simulink model "proc_control_node"  (R2020a)
settings: Solver=FixedStepAuto  StartTime=0.0  StopTime=inf  FixedStep=.005  RelTol=1e-3
model workspace (MAT data in the model file):
  SL_ROS_VariableLengthArrays_MaxSizes.CommonInfo.ArrayTruncateAction = 'EmitWarning'
  SL_ROS_VariableLengthArrays_MaxSizes.MsgTypeMap = containers.Map
  SL_ROS_VariableLengthArrays_MaxSizes.MsgTypeMap.serialization.keys = {}
  SL_ROS_VariableLengthArrays_MaxSizes.MsgTypeMap.serialization.values = {}
  SL_ROS_VariableLengthArrays_MaxSizes.MsgTypeMap.serialization.uniformity = 0
  SL_ROS_VariableLengthArrays_MaxSizes.MsgTypeMap.serialization.keyType = 'char'
  SL_ROS_VariableLengthArrays_MaxSizes.MsgTypeMap.serialization.valueType = 'any'
undefined symbols (not defined in the file): InitController
libraries: robotlib x6, simulink x1
settings Model: SimulationMode=accelerator  PauseTimes=1000  Creator=Lamarre  LastModifiedBy=lamarre
settings OptimizationCC: EnhancedBackFolding=on  PassReuseOutputArgsAs=Individual arguments  ZeroExternalMemoryAtStartup=off  ZeroInternalMemoryAtStartup=off  MaxStackSize=64  OptimizeBlockOrder=speed  DifferentSizesBufferReuse=on  OptimizationCustomize=off  EfficientTunableParamExpr=on
settings DebuggingCC: ParameterTunabilityLossMsg=error  FcnCallInpInsideContextMsg=warning  UnderSpecifiedDimensionMsg=warning
settings HardwareCC: ProdBitPerPointer=32  ProdBitPerSizeT=32  ProdBitPerPtrDiffT=32  ProdLargestAtomicInteger=Long  ProdWordSize=32  ProdHWDeviceType=ARM Compatible->ARM 8
settings ModelReferenceCC: ModelReferenceNumInstancesAllowed=Single
settings SFSimCC: MATLABDynamicMemAlloc=off
settings RTWCC: SystemTargetFile=ert.tlc  HardwareBoard=Robot Operating System (ROS)  TemplateMakefile=ert_default_tmf  Toolchain=Catkin  BuildConfiguration=Faster Runs  TargetLang=C++
settings CodeAppCC: ForceParamTrailComments=on  IgnoreCustomStorageClasses=off  OperatorAnnotations=on  SimulinkDataObjDesc=on  SFDataObjDesc=on  InsertBlockDesc=on
settings ERTTargetCC: SupportContinuousTime=on  SupportVariableSizeSignals=on  TargetOS=NativeThreadsExample  MultiInstanceErrorCode=Warning  RootIOFormat=Structure reference

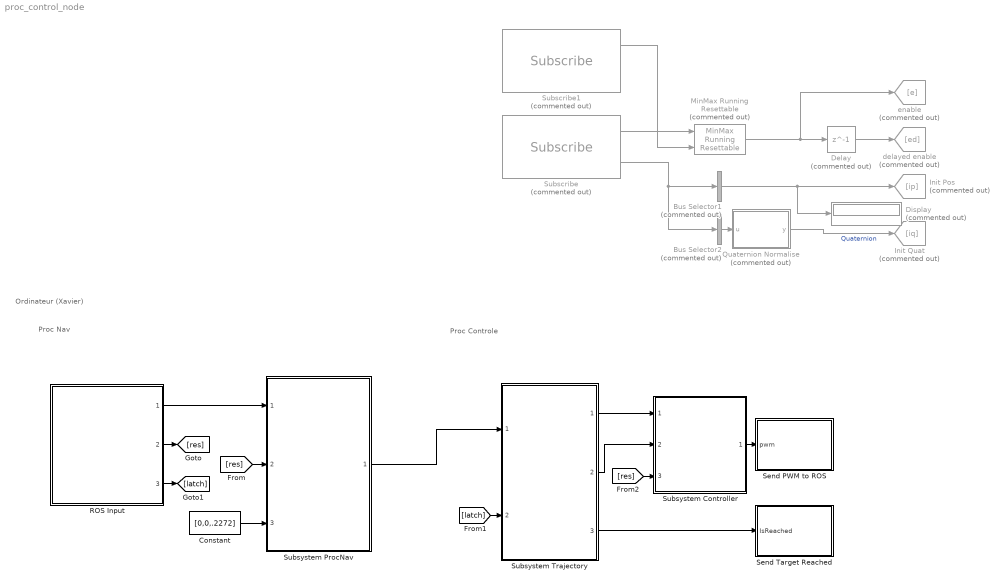
== system proc_control_node ==
  note: Proc Nav
  note: Proc Controle
  note: Ordinateur (Xavier)
  " Init Pos" : Goto  Commented=on  GotoTag=ip
  " Init Quat" : Goto  Commented=on  GotoTag=iq
  " enable" : Goto  Commented=on  GotoTag=e
  Bus Selector1 : BusSelector  Commented=on  OutputSignals=Position.X,Position.Y,Position.Z  OutputAsBus=on
  Bus Selector2 : BusSelector  Commented=on  OutputSignals=Orientation.W,Orientation.Z,Orientation.Y,Orientation.X  OutputAsBus=on
  Constant : Constant  Value=[0,0,.2272]
  Delay : Delay  Commented=on  DelayLength=1
  Display : Display  Commented=on
  MinMax Running Resettable : simulink/Math Operations/MinMax Running Resettable  Commented=on  Function=max  vinit=0.0
  Quaternion Normalise : MATLAB Function  Commented=on  TreatAsAtomicUnit=on
  ROS Input : Subsystem  ReferencedSubsystem=proc_nav_ros_input
  Send PWM to ROS : Subsystem
  "Send Target Reached " : Subsystem
  Subscribe : robotlib/Subscribe  Commented=on  topicSource=Specify your own  topic=/proc_control/start  messageType=geometry_msgs/Pose  sampleTime=-1  messageQueueLength=1
  Subscribe1 : robotlib/Subscribe  Commented=on  topicSource=Specify your own  topic=/proc_control/kill  messageType=std_msgs/Bool  sampleTime=-1  messageQueueLength=1
  Subsystem Controller : Subsystem  InitFcn=InitController;  ReferencedSubsystem=Controller
  Subsystem ProcNav : Subsystem  ReferencedSubsystem=ProcNav
  Subsystem Trajectory : Subsystem  InitFcn=|  ReferencedSubsystem=Trajectory
      | InitTrajectory
      | %trajec;
  delayed enable : Goto  Commented=on  GotoTag=ed
  wires:
  Subsystem ProcNav/1 -> Subsystem Trajectory/1
  Subsystem Trajectory/1 -> Subsystem Controller/1
  Constant/1 -> Subsystem ProcNav/3
  Subsystem Trajectory/2 -> Subsystem Controller/2
  Subsystem Trajectory/3 -> "Send Target Reached "/1(IsReached)
  MinMax Running Resettable/1 -> " enable"/1, Delay/1
  Subscribe/1 -> MinMax Running Resettable/1
  Subscribe/2 -> Bus Selector2/1, Bus Selector1/1
  Delay/1 -> delayed enable/1
  Bus Selector1/1 -> Display/1, " Init Pos"/1
  Subscribe1/1 -> MinMax Running Resettable/2
  Bus Selector2/1 -> Quaternion Normalise/1(u)
  Quaternion Normalise/1(y) -> " Init Quat"/1  "Quaternion"
  Subsystem Controller/1 -> Send PWM to ROS/1(pwm)
  ROS Input/1 -> Subsystem ProcNav/1
  ROS Input/2 -> [res]
  [res] -> Subsystem ProcNav/2
  [latch] -> Subsystem Trajectory/2
  [res] -> Subsystem Controller/3
  ROS Input/3 -> [latch]

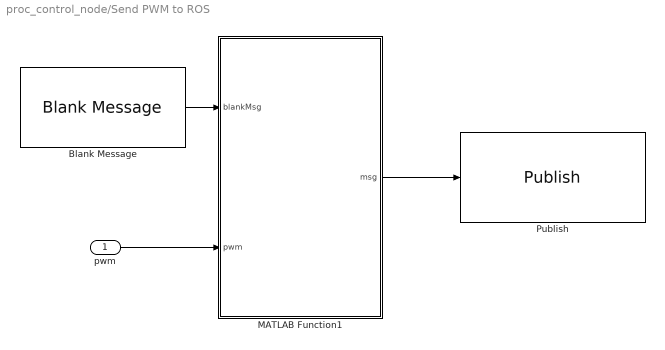
== system proc_control_node/Send PWM to ROS ==
  pwm : Inport
  Blank Message : robotlib/Blank Message  messageClass=Message  entityType=std_msgs/UInt16MultiArray  messageType=std_msgs/UInt16MultiArray  SampleTime=inf
  MATLAB Function1 : MATLAB Function  TreatAsAtomicUnit=on
  Publish : robotlib/Publish  topicSource=Specify your own  topic=/provider_thruster/thruster_pwm  messageType=std_msgs/UInt16MultiArray  messageQueueLength=1
  wires:
  MATLAB Function1/1(msg) -> Publish/1
  Blank Message/1 -> MATLAB Function1/1(blankMsg)
  pwm/1 -> MATLAB Function1/2(pwm)

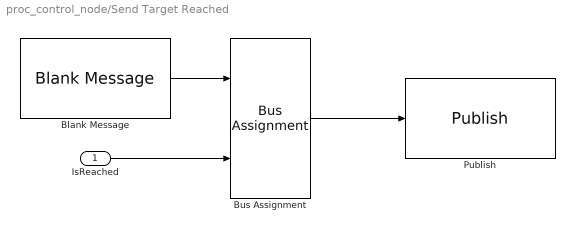
== system proc_control_node/Send Target Reached  ==
  IsReached : Inport
  Blank Message : robotlib/Blank Message  messageClass=Message  entityType=std_msgs/Bool  messageType=std_msgs/Bool  SampleTime=inf
  Bus Assignment : BusAssignment  AssignedSignals=Data
  Publish : robotlib/Publish  topicSource=Specify your own  topic=proc_control_matlab/target_reached  messageType=std_msgs/Bool  messageQueueLength=1
  wires:
  Blank Message/1 -> Bus Assignment/1
  IsReached/1 -> Bus Assignment/2
  Bus Assignment/1 -> Publish/1

== matlab function proc_control_node/Send PWM to ROS/MATLAB Function1 ==
  data: blankMsg input; pwm input; msg output Bus: SL_Bus_proc_control_node_std_msgs_UInt16MultiArray
function msg = assignThrusterPwm(blankMsg, pwm)
msg = blankMsg;
msg.Data(1:8) = cast(pwm, 'uint16');
msg.Data_SL_Info.CurrentLength = uint32(8);

== matlab function proc_control_node/Quaternion Normalise ==
  data: u input size=4; y output size=4
function y = Normalize(u)
%Normailse le quaternions pour éviter la distortions crée par l'erreur de
% de l'intégration.
d=norm(u);
n=u/d;
if isnan(n)
    y=[1;0;0;0];
else
    y = n;
end
